simulink model "assignment_1"  (R2020b)
settings: Solver=VariableStepAuto  StartTime=0.0  StopTime=100  RelTol=1e-3
values from neighbouring files (symbols this model uses):
  b = 50    [values.m]
  k1 = 50    [values.m]
  k12 = 200    [values.m]
  M1 = 100    [values.m]
  M2 = 100    [values.m]
settings Model: Creator=Sudhanshu  LastModifiedBy=Sudhanshu

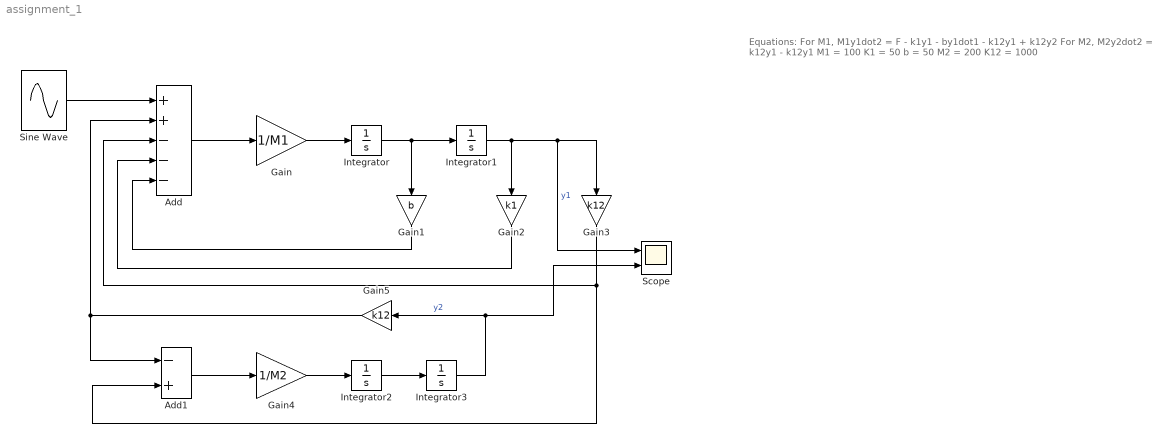
== system assignment_1 ==
  note: Equations:
      |
      | For M1,
      | M1y1dot2 = F - k1y1 - by1dot1 - k12y1 + k12y2
      |
      | For M2,
      | M2y2dot2 = k12y1 - k12y1
      |
      | M1 = 100
      | K1 = 50
      | b = 50
      |
      | M2 = 200
      | K12 = 1000
  Add : Sum  Inputs=++---
  Add1 : Sum  Inputs=-+
  Gain : Gain  Gain=1/M1
  Gain1 : Gain  Gain=b
  Gain2 : Gain  Gain=k1
  Gain3 : Gain  Gain=k12
  Gain4 : Gain  Gain=1/M2
  Gain5 : Gain  Gain=k12
  Integrator{,1..3} (4 alike) : Integrator
  Scope : Scope  NumInputPorts=2
  Sine Wave : Sin  Amplitude=2  Frequency=10  SampleTime=0
  wires:
  Gain/1 -> Integrator/1
  Sine Wave/1 -> Add/1
  Add/1 -> Gain/1
  Integrator/1 -> Integrator1/1, Gain1/1
  Integrator1/1 -> Gain3/1, Scope/1, Gain2/1  "y1"
  Gain1/1 -> Add/5
  Gain2/1 -> Add/4
  Gain3/1 -> Add1/2, Add/3
  Gain4/1 -> Integrator2/1
  Integrator2/1 -> Integrator3/1
  Integrator3/1 -> Scope/2, Gain5/1  "y2"
  Gain5/1 -> Add1/1, Add/2
  Add1/1 -> Gain4/1
